simulink subsystem "Guidance_SubSystem"  (R2022b)
settings: Solver=VariableStepAuto  StartTime=0.0  StopTime=10.0  RelTol=1e-3
settings Model: Creator=Wikian  LastModifiedBy=Wikian

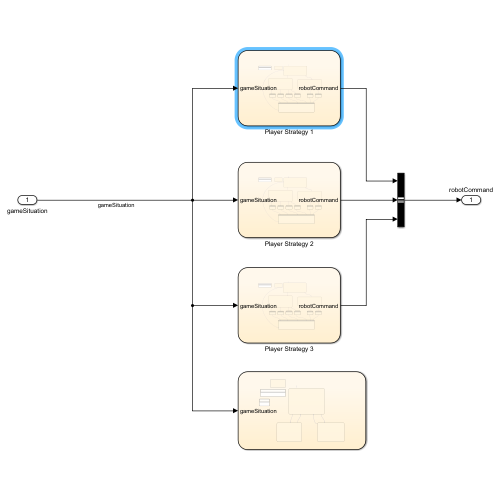
[thumbnail: Simulink's stored preview of the top-level diagram]
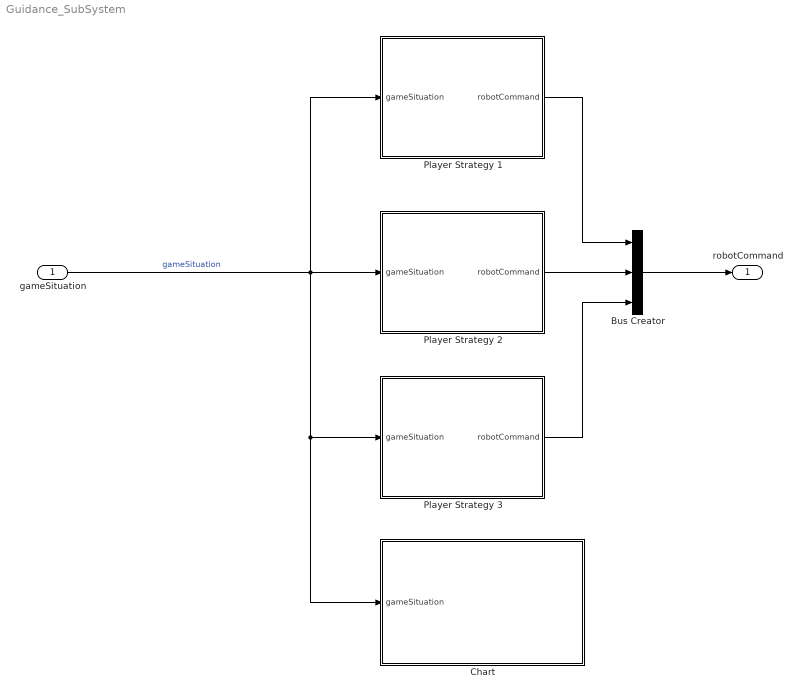
== system Guidance_SubSystem ==
  gameSituation : Inport
  Bus Creator : BusCreator  Inputs=3
  Chart : Stateflow chart  TreatAsAtomicUnit=on
  Player Strategy 1 : Stateflow chart  TreatAsAtomicUnit=on
  Player Strategy 2 : Stateflow chart  TreatAsAtomicUnit=on
  Player Strategy 3 : Stateflow chart  TreatAsAtomicUnit=on
  robotCommand : Outport
  wires:
  Bus Creator/1 -> robotCommand/1
  Player Strategy 2/1(robotCommand) -> Bus Creator/2
  Player Strategy 1/1(robotCommand) -> Bus Creator/1
  gameSituation/1 -> Player Strategy 2/1(gameSituation), Player Strategy 1/1(gameSituation), Chart/1(gameSituation), Player Strategy 3/1(gameSituation)  "gameSituation"
  Player Strategy 3/1(robotCommand) -> Bus Creator/3

== stateflow chart Guidance_SubSystem/Player Strategy 1 ==
  state ROBOT 1 [group]
    (Strategy for robot 1~3)
  state InitialState
    en:
    if gameSituation.kickConfirmation == true
    robotCommand.kick = false;
    end
    du:
    id = 1 % Team1(Home) Robot 1
    shootDistThres = 2.5;
    kickableAreaRadius = 0.1;
    homeGoalPose = [4.5, 0];
    awayGoalPose = [-4.5, 0];
    homeAttackPositions = [[2.5,0,0]; [1,2,0]; [1,-2,0]];
    homeDefendPositions = [[-2,0,0]; [-3,2,0]; [-3,-2,0]];
    ex:
  state Attack
    en:
    %%calculate the distance to the goal
    teamDistToGoal = [];
    for idx=1:1:3
    teamDistToGoal(idx) = distTo(gameSituation.robotCurrentPose(idx,1:2) - awayGoalPose);
    end
    distToGoal1 = distTo(gameSituation.robotCurrentPose(id,1:2) - awayGoalPose);
    du:
    %calculate the distance to the ball
    teamDistToBall = [];
    for idx=1:1:3
    teamDistToBall(idx) = distTo(gameSituation.robotCurrentPose(idx,1:2) - ...
    gameSituation.ballCurrentPose(1:2));
    end
    distToBall = distTo(gameSituation.robotCurrentPose(id,1:2) - ...
    gameSituation.ballCurrentPose(1:2))
  state Defend
    en:
    %%calculate the distance to the home goal
    teamDistToOwnGoal = [];
    for idx=1:1:3
    teamDistToOwnGoal = distToGoal(gameSituation.robotCurrentPose(idx,1:2) - homeGoalPose);
    end
    distToOwnGoal = distToGoal(gameSituation.robotCurrentPose(id,1:2) - homeGoalPose);
    du:
    ex:
  state Position
    en:
    playerAttackPosition = homeAttackPositions(id, :);
    kickPower = 1;
    kickState = false;
    du:
    desiredPosition = player1AttackPosition;
    ex:
    isdone = true;
  state Shoot
    en:
    angleBallGoal = atan2d(awayGoalPosition(2) - gameSituation.ballCurrentPose(2), ...
    awayGoalPosition(1) - gameSituation.ballCurrentPose(1));
    kickPower = 100;
    kickState = true;
    kickDirection = 180 + angleBallGoal;
    du:
    desiredPosition = [gameSituation.ballCurrentPose(1) + cosd(angleBallGoal) * kickableAreaRadius, ...
    gameSituation.ballCurrentPose(2) + sind(angleBallGoal) * kickableAreaRadius];
    ex:
    isdone = true;
  state Intercept
    en:
    angleBallGoal = atan2d(awayGoalPosition(2) - gameSituation.ballCurrentPose(2), ...
    awayGoalPosition(1) - gameSituation.ballCurrentPose(1));
    kickPower = 50;
    kickState = true;
    kickDirection = 180 + angleBallGoal;
    du:
    desiredPosition = [gameSituation.ballCurrentPose(1) + cosd(angleBallGoal) * kickableAreaRadius, ...
    gameSituation.ballCurrentPose(2) + sind(angleBallGoal) * kickableAreaRadius];
    ex:
    isdone = true;
  state Formation
    en:
    playerDefendPosition = homeDefendPositions(id, :);
    kickPower = 1;
    kickState = false;
    desiredPosition = playerDefendPosition;
    ex:
    isdone = true;
  state Pass
    en:
    [minval,minidx] = min(teamDistToGoal)
    angleBallPlayer = atan2d(gameSituation.robotCurrentPose(minidx, 2) - gameSituation.ballCurrentPose(2), ...
    gameSituation.robotCurrentPose(minidx, 1) - gameSituation.ballCurrentPose(1));
    kickPower = 66;
    kickState = true;
    kickDirection = 180 + angleBallPlayer;
    du:
    desiredPosition = [gameSituation.ballCurrentPose(1) + cosd(angleBallPlayer) * kickableAreaRadius, ...
    gameSituation.ballCurrentPose(2) + sind(angleBallPlayer) * kickableAreaRadius];
    ex:
    isdone = true;
  state Dribble
    en:
    angleBallGoal = atan2d(awayGoalPosition(2) - gameSituation.ballCurrentPose(2), ...
    awayGoalPosition(1) - gameSituation.ballCurrentPose(1));
    kickPower = 33;
    %%should be designed as the kickPower = kickPowerCofficent * 100
    %%kickPowerCofficieant should also be calculated by distance
    kickState = true;
    kickDirection = 180 + angleBallGoal;
    du:
    desiredPosition = [gameSituation.ballCurrentPose(1) + cosd(angleBallGoal) * kickableAreaRadius, ...
    gameSituation.ballCurrentPose(2) + sind(angleBallGoal) * kickableAreaRadius];
    ex:
    isdone = true;
  state Kick
    state MoveTo1
      en: isdone = false;
      du:
      robotCommand.robotDestinationPose = [desiredPosition, kickDirection];
      ex:
    state KickTo
      en:
      robotCommand.kick = kickState;
      robotCommand.kickProperty = kickPower;
      du:
      ex:
    MoveTo1 -> KickTo : [gameSituation.robotCurrentPose == robotCommand.DestinationPose]
  Position -> MoveTo1 : [isdone]
  Formation -> MoveTo1 : [isdone]
  Intercept -> MoveTo1 : [isdone]
  KickTo -> InitialState : [after(1,sec)]
  Pass -> MoveTo1 : [isdone]
  Shoot -> MoveTo1 : [isdone]
  Dribble -> MoveTo1 : [isdone]
  (default) -> InitialState
  InitialState -> Attack [order 2] : [gameSituation.ballLastCommandBy(1) == 1]
  InitialState -> Defend [order 1] : [gameSituation.ballLastCommandBy(1) == 2]
  Defend -> Intercept [order 1] : [distToOwnGoal ~= max(teamDistToOwnGoal)]
  Defend -> Formation [order 2] : [distToOwnGoal == max(teamDistToOwnGoal)]
  Attack -> Pass [order 3] : [distToGoal1 ~= min(teamDistToGoal)&& distToBall == min(teamDistToBall)]
  Attack -> Dribble [order 4] : [distToBall == min(teamDistToBall) && distToGoal1 == min(teamDistToGoal) && distToGoal1 > shootDistThres]
  Attack -> Shoot [order 2] : [distToBall == min(teamDistToBall) && distToGoal1 == min(teamDistToGoal) && distToGoal1 < shootDistThres]
  Attack -> Position [order 1] : [distToBall ~= min(teamDistToBall)]
  data: robotPosition function_input; goalPosition function_input; dist function_output; awayGoalPose local; homeGoalPose local; id local; idx local; angleBallGoal local; desiredPosition local; distToOwnGoal local; kickDirection local; kickPower local; kickState local; minidx local; playerDefendPosition local; teamDistToGoal local; teamDistToOwnGoal local; minval local; isdone local boolean =false; playerAttackPosition local; shootDistThres parameter; awayGoalPosition local; player1AttackPosition local; gameSituation input Bus: gameSituation; kickableAreaRadius local; distToGoal1 local; angleBallPlayer local; robotCommand output Bus: robotCommand; distToBall local; teamDistToBall local; homeAttackPositions local; homeDefendPositions local
  function dist = distTo(robotPosition,goalPosition):
    | function dist = distTo(robotPosition,goalPosition)
    |     dist = norm(robotPosition - goalPosition);
    | end

== stateflow chart Guidance_SubSystem/Player Strategy 2 ==
  state ROBOT 1 [group]
    (Strategy for robot 1~3)
  state InitialState
    en:
    if gameSituation.kickConfirmation == true
    robotCommand.kick = false;
    end
    du:
    id = 2 % Team1(Home) Robot 1
    shootDistThres = 2.5;
    kickableAreaRadius = 0.1;
    homeGoalPose = [4.5, 0];
    awayGoalPose = [-4.5, 0];
    homeAttackPositions = [[2.5,0,0]; [1,2,0]; [1,-2,0]];
    homeDefendPositions = [[-2,0,0]; [-3,2,0]; [-3,-2,0]];
    ex:
  state Attack
    en:
    %%calculate the distance to the goal
    teamDistToGoal = [];
    for idx=1:1:3
    teamDistToGoal(idx) = distTo(gameSituation.robotCurrentPose(idx,1:2) - awayGoalPose);
    end
    distToGoal1 = distTo(gameSituation.robotCurrentPose(id,1:2) - awayGoalPose);
    du:
    %calculate the distance to the ball
    teamDistToBall = [];
    for idx=1:1:3
    teamDistToBall(idx) = distTo(gameSituation.robotCurrentPose(idx,1:2) - ...
    gameSituation.ballCurrentPose(1:2));
    end
    distToBall = distTo(gameSituation.robotCurrentPose(id,1:2) - ...
    gameSituation.ballCurrentPose(1:2))
  state Defend
    en:
    %%calculate the distance to the home goal
    teamDistToOwnGoal = [];
    for idx=1:1:3
    teamDistToOwnGoal = distToGoal(gameSituation.robotCurrentPose(idx,1:2) - homeGoalPose);
    end
    distToOwnGoal = distToGoal(gameSituation.robotCurrentPose(id,1:2) - homeGoalPose);
    du:
    ex:
  state Position
    en:
    playerAttackPosition = homeAttackPositions(id, :);
    kickPower = 1;
    kickState = false;
    du:
    desiredPosition = player1AttackPosition;
    ex:
    isdone = true;
  state Shoot
    en:
    angleBallGoal = atan2d(awayGoalPosition(2) - gameSituation.ballCurrentPose(2), ...
    awayGoalPosition(1) - gameSituation.ballCurrentPose(1));
    kickPower = 100;
    kickState = true;
    kickDirection = 180 + angleBallGoal;
    du:
    desiredPosition = [gameSituation.ballCurrentPose(1) + cosd(angleBallGoal) * kickableAreaRadius, ...
    gameSituation.ballCurrentPose(2) + sind(angleBallGoal) * kickableAreaRadius];
    ex:
    isdone = true;
  state Intercept
    en:
    angleBallGoal = atan2d(awayGoalPosition(2) - gameSituation.ballCurrentPose(2), ...
    awayGoalPosition(1) - gameSituation.ballCurrentPose(1));
    kickPower = 50;
    kickState = true;
    kickDirection = 180 + angleBallGoal;
    du:
    desiredPosition = [gameSituation.ballCurrentPose(1) + cosd(angleBallGoal) * kickableAreaRadius, ...
    gameSituation.ballCurrentPose(2) + sind(angleBallGoal) * kickableAreaRadius];
    ex:
    isdone = true;
  state Formation
    en:
    playerDefendPosition = homeDefendPositions(id, :);
    kickPower = 1;
    kickState = false;
    desiredPosition = playerDefendPosition;
    ex:
    isdone = true;
  state Pass
    en:
    [minval,minidx] = min(teamDistToGoal)
    angleBallPlayer = atan2d(gameSituation.robotCurrentPose(minidx, 2) - gameSituation.ballCurrentPose(2), ...
    gameSituation.robotCurrentPose(minidx, 1) - gameSituation.ballCurrentPose(1));
    kickPower = 66;
    kickState = true;
    kickDirection = 180 + angleBallPlayer;
    du:
    desiredPosition = [gameSituation.ballCurrentPose(1) + cosd(angleBallPlayer) * kickableAreaRadius, ...
    gameSituation.ballCurrentPose(2) + sind(angleBallPlayer) * kickableAreaRadius];
    ex:
    isdone = true;
  state Dribble
    en:
    angleBallGoal = atan2d(awayGoalPosition(2) - gameSituation.ballCurrentPose(2), ...
    awayGoalPosition(1) - gameSituation.ballCurrentPose(1));
    kickPower = 33;
    %%should be designed as the kickPower = kickPowerCofficent * 100
    %%kickPowerCofficieant should also be calculated by distance
    kickState = true;
    kickDirection = 180 + angleBallGoal;
    du:
    desiredPosition = [gameSituation.ballCurrentPose(1) + cosd(angleBallGoal) * kickableAreaRadius, ...
    gameSituation.ballCurrentPose(2) + sind(angleBallGoal) * kickableAreaRadius];
    ex:
    isdone = true;
  state Kick
    state MoveTo1
      en: isdone = false;
      du:
      robotCommand.robotDestinationPose = [desiredPosition, kickDirection];
      ex:
    state KickTo
      en:
      robotCommand.kick = kickState;
      robotCommand.kickProperty = kickPower;
      du:
      ex:
    MoveTo1 -> KickTo : [gameSituation.robotCurrentPose == robotCommand.DestinationPose]
  Position -> MoveTo1 : [isdone]
  Formation -> MoveTo1 : [isdone]
  Intercept -> MoveTo1 : [isdone]
  KickTo -> InitialState : [after(1,sec)]
  Pass -> MoveTo1 : [isdone]
  Shoot -> MoveTo1 : [isdone]
  Dribble -> MoveTo1 : [isdone]
  (default) -> InitialState
  InitialState -> Attack [order 2] : [gameSituation.ballLastCommandBy(1) == 1]
  InitialState -> Defend [order 1] : [gameSituation.ballLastCommandBy(1) == 2]
  Defend -> Intercept [order 1] : [distToOwnGoal ~= max(teamDistToOwnGoal)]
  Defend -> Formation [order 2] : [distToOwnGoal == max(teamDistToOwnGoal)]
  Attack -> Pass [order 3] : [distToGoal1 ~= min(teamDistToGoal)&& distToBall == min(teamDistToBall)]
  Attack -> Dribble [order 4] : [distToBall == min(teamDistToBall) && distToGoal1 == min(teamDistToGoal) && distToGoal1 > shootDistThres]
  Attack -> Shoot [order 2] : [distToBall == min(teamDistToBall) && distToGoal1 == min(teamDistToGoal) && distToGoal1 < shootDistThres]
  Attack -> Position [order 1] : [distToBall ~= min(teamDistToBall)]
  data: robotPosition function_input; goalPosition function_input; dist function_output; awayGoalPose local; homeGoalPose local; id local; idx local; angleBallGoal local; desiredPosition local; distToOwnGoal local; kickDirection local; kickPower local; kickState local; minidx local; playerDefendPosition local; teamDistToGoal local; teamDistToOwnGoal local; minval local; isdone local boolean =false; playerAttackPosition local; shootDistThres parameter; awayGoalPosition local; player1AttackPosition local; gameSituation input Bus: gameSituation; kickableAreaRadius local; distToGoal1 local; angleBallPlayer local; robotCommand output Bus: robotCommand; distToBall local; teamDistToBall local; homeAttackPositions local; homeDefendPositions local
  function dist = distTo(robotPosition,goalPosition):
    | function dist = distTo(robotPosition,goalPosition)
    |     dist = norm(robotPosition - goalPosition);
    | end

== stateflow chart Guidance_SubSystem/Player Strategy 3 ==
  state InitialState
    en:
    if gameSituation.kickConfirmation == true
    robotCommand.kick = false;
    end
    du:
    id = 3 % Team1(Home) Robot 1
    shootDistThres = 2.5;
    kickableAreaRadius = 0.1;
    homeGoalPose = [4.5, 0];
    awayGoalPose = [-4.5, 0];
    homeAttackPositions = [[2.5,0,0]; [1,2,0]; [1,-2,0]];
    homeDefendPositions = [[-2,0,0]; [-3,2,0]; [-3,-2,0]];
    ex:
  state ROBOT 1 [group]
    (Strategy for robot 1~3)
  state Attack
    en:
    %%calculate the distance to the goal
    teamDistToGoal = [];
    for idx=1:1:3
    teamDistToGoal(idx) = distTo(gameSituation.robotCurrentPose(idx,1:2) - awayGoalPose);
    end
    distToGoal1 = distTo(gameSituation.robotCurrentPose(id,1:2) - awayGoalPose);
    du:
    %calculate the distance to the ball
    teamDistToBall = [];
    for idx=1:1:3
    teamDistToBall(idx) = distTo(gameSituation.robotCurrentPose(idx,1:2) - ...
    gameSituation.ballCurrentPose(1:2));
    end
    distToBall = distTo(gameSituation.robotCurrentPose(id,1:2) - ...
    gameSituation.ballCurrentPose(1:2))
  state Defend
    en:
    %%calculate the distance to the home goal
    teamDistToOwnGoal = [];
    for idx=1:1:3
    teamDistToOwnGoal = distToGoal(gameSituation.robotCurrentPose(idx,1:2) - homeGoalPose);
    end
    distToOwnGoal = distToGoal(gameSituation.robotCurrentPose(id,1:2) - homeGoalPose);
    du:
    ex:
  state Position
    en:
    playerAttackPosition = homeAttackPositions(id, :);
    kickPower = 1;
    kickState = false;
    du:
    desiredPosition = player1AttackPosition;
    ex:
    isdone = true;
  state Shoot
    en:
    angleBallGoal = atan2d(awayGoalPosition(2) - gameSituation.ballCurrentPose(2), ...
    awayGoalPosition(1) - gameSituation.ballCurrentPose(1));
    kickPower = 100;
    kickState = true;
    kickDirection = 180 + angleBallGoal;
    du:
    desiredPosition = [gameSituation.ballCurrentPose(1) + cosd(angleBallGoal) * kickableAreaRadius, ...
    gameSituation.ballCurrentPose(2) + sind(angleBallGoal) * kickableAreaRadius];
    ex:
    isdone = true;
  state Intercept
    en:
    angleBallGoal = atan2d(awayGoalPosition(2) - gameSituation.ballCurrentPose(2), ...
    awayGoalPosition(1) - gameSituation.ballCurrentPose(1));
    kickPower = 50;
    kickState = true;
    kickDirection = 180 + angleBallGoal;
    du:
    desiredPosition = [gameSituation.ballCurrentPose(1) + cosd(angleBallGoal) * kickableAreaRadius, ...
    gameSituation.ballCurrentPose(2) + sind(angleBallGoal) * kickableAreaRadius];
    ex:
    isdone = true;
  state Formation
    en:
    playerDefendPosition = homeDefendPositions(id, :);
    kickPower = 1;
    kickState = false;
    desiredPosition = playerDefendPosition;
    ex:
    isdone = true;
  state Pass
    en:
    [minval,minidx] = min(teamDistToGoal)
    angleBallPlayer = atan2d(gameSituation.robotCurrentPose(minidx, 2) - gameSituation.ballCurrentPose(2), ...
    gameSituation.robotCurrentPose(minidx, 1) - gameSituation.ballCurrentPose(1));
    kickPower = 66;
    kickState = true;
    kickDirection = 180 + angleBallPlayer;
    du:
    desiredPosition = [gameSituation.ballCurrentPose(1) + cosd(angleBallPlayer) * kickableAreaRadius, ...
    gameSituation.ballCurrentPose(2) + sind(angleBallPlayer) * kickableAreaRadius];
    ex:
    isdone = true;
  state Dribble
    en:
    angleBallGoal = atan2d(awayGoalPosition(2) - gameSituation.ballCurrentPose(2), ...
    awayGoalPosition(1) - gameSituation.ballCurrentPose(1));
    kickPower = 33;
    %%should be designed as the kickPower = kickPowerCofficent * 100
    %%kickPowerCofficieant should also be calculated by distance
    kickState = true;
    kickDirection = 180 + angleBallGoal;
    du:
    desiredPosition = [gameSituation.ballCurrentPose(1) + cosd(angleBallGoal) * kickableAreaRadius, ...
    gameSituation.ballCurrentPose(2) + sind(angleBallGoal) * kickableAreaRadius];
    ex:
    isdone = true;
  state Kick
    state MoveTo1
      en: isdone = false;
      du:
      robotCommand.robotDestinationPose = [desiredPosition, kickDirection];
      ex:
    state KickTo
      en:
      robotCommand.kick = kickState;
      robotCommand.kickProperty = kickPower;
      du:
      ex:
    MoveTo1 -> KickTo : [gameSituation.robotCurrentPose == robotCommand.DestinationPose]
  Position -> MoveTo1 : [isdone]
  Formation -> MoveTo1 : [isdone]
  Intercept -> MoveTo1 : [isdone]
  KickTo -> InitialState : [after(1,sec)]
  Pass -> MoveTo1 : [isdone]
  Shoot -> MoveTo1 : [isdone]
  Dribble -> MoveTo1 : [isdone]
  (default) -> InitialState
  InitialState -> Attack [order 2] : [gameSituation.ballLastCommandBy(1) == 1]
  InitialState -> Defend [order 1] : [gameSituation.ballLastCommandBy(1) == 2]
  Defend -> Intercept [order 1] : [distToOwnGoal ~= max(teamDistToOwnGoal)]
  Defend -> Formation [order 2] : [distToOwnGoal == max(teamDistToOwnGoal)]
  Attack -> Pass [order 3] : [distToGoal1 ~= min(teamDistToGoal)&& distToBall == min(teamDistToBall)]
  Attack -> Dribble [order 4] : [distToBall == min(teamDistToBall) && distToGoal1 == min(teamDistToGoal) && distToGoal1 > shootDistThres]
  Attack -> Shoot [order 2] : [distToBall == min(teamDistToBall) && distToGoal1 == min(teamDistToGoal) && distToGoal1 < shootDistThres]
  Attack -> Position [order 1] : [distToBall ~= min(teamDistToBall)]
  data: robotPosition function_input; goalPosition function_input; dist function_output; awayGoalPose local; homeGoalPose local; id local; idx local; angleBallGoal local; desiredPosition local; distToOwnGoal local; kickDirection local; kickPower local; kickState local; minidx local; playerDefendPosition local; teamDistToGoal local; teamDistToOwnGoal local; minval local; isdone local boolean =false; playerAttackPosition local; shootDistThres parameter; awayGoalPosition local; player1AttackPosition local; gameSituation input Bus: gameSituation; kickableAreaRadius local; distToGoal1 local; angleBallPlayer local; robotCommand output Bus: robotCommand; distToBall local; teamDistToBall local; homeAttackPositions local; homeDefendPositions local
  function dist = distTo(robotPosition,goalPosition):
    | function dist = distTo(robotPosition,goalPosition)
    |     dist = norm(robotPosition - goalPosition);
    | end

== stateflow chart Guidance_SubSystem/Chart ==
  state ROBOT 1 [group]
    (Strategy for robot 1~3)
  state initialState
    en:
    if gameSituation.kickConfirmation == true
    robotCommand.kick = false;
    end
    du:
    id = 3 % Team1(Home) Robot 1
    shootDistThres = 2.5;
    kickableAreaRadius = 0.1;
    homeGoalPose = [5, 0];
    awayGoalPose = [-5, 0];
    homeAttackPositions = [[2.5,0,0]; [1,2,0]; [1,-2,0]];
    homeDefendPositions = [[-2,0,0]; [-3,2,0]; [-3,-2,0]];
    ex:
    distToBall = distTo(gameSituation.robotCurrentPose(id,1:2) - ...
    gameSituation.ballCurrentPose(1:2))
  state Dive
  state Position
  (default) -> initialState
  initialState -> Dive [order 1] : [gameSituation.ballLastCommandBy(1) == 2]
  Dive -> initialState
  Position -> initialState
  initialState -> Position [order 2]
  data: robotPosition function_input; goalPosition function_input; dist function_output; gameSituation input
  function dist = distTo(robotPosition,goalPosition):
    | function dist = distTo(robotPosition,goalPosition)
    |     dist = norm(robotPosition - goalPosition);
    | end
  function ?:
    | function
